simulink model "Model_zawieszenia"  (R2024b)
settings: Solver=VariableStepAuto  StartTime=0.0  StopTime=10.0  RelTol=1e-3
model workspace (MAT data in the model file):
  F = 1000
  alpha_zaw = 500
  c_zaw = 400
  m = 1000
settings Model: Creator=mati  LastModifiedBy=mati

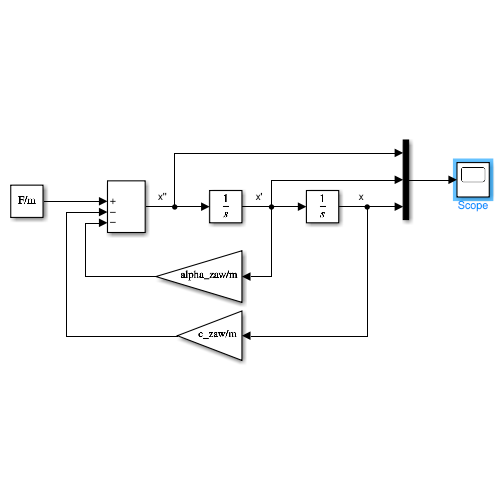
[thumbnail: Simulink's stored preview of the top-level diagram]
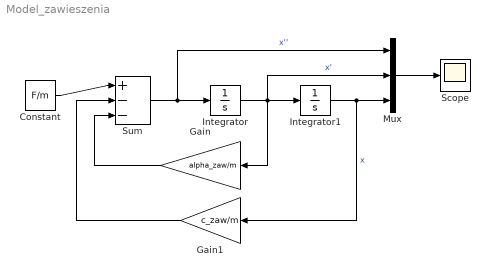
== system Model_zawieszenia ==
  Constant : Constant  Value=F/m
  Gain : Gain  Gain=alpha_zaw/m
  Gain1 : Gain  Gain=c_zaw/m
  Integrator : Integrator
  Integrator1 : Integrator  InitialCondition=1
  Mux : Mux  Inputs=3
  Scope : Scope
  Sum : Sum  Inputs=|+--
  wires:
  Sum/1 -> Integrator/1, Mux/1  "x''"
  Gain/1 -> Sum/3
  Integrator/1 -> Integrator1/1, Mux/2, Gain/1  "x'"
  Integrator1/1 -> Mux/3, Gain1/1  "x"
  Gain1/1 -> Sum/2
  Constant/1 -> Sum/1
  Mux/1 -> Scope/1
